simulink model "PID_simulink"  (R2018a)
settings: Solver=FixedStepAuto  StartTime=0.0  StopTime=t_end  FixedStep=0.0001  MinStep=1e-4  RelTol=1e-3
values from neighbouring files (symbols this model uses):
  Den = [1 12 24]    [PID.m]
  Kd = 3    [PID.m]
  Ki = 70    [PID.m]
  Kp = 50    [PID.m]
  Num = [2]    [PID.m]
settings Model: Creator=Milosh Yokich  LastModifiedBy=Milosh Yokich

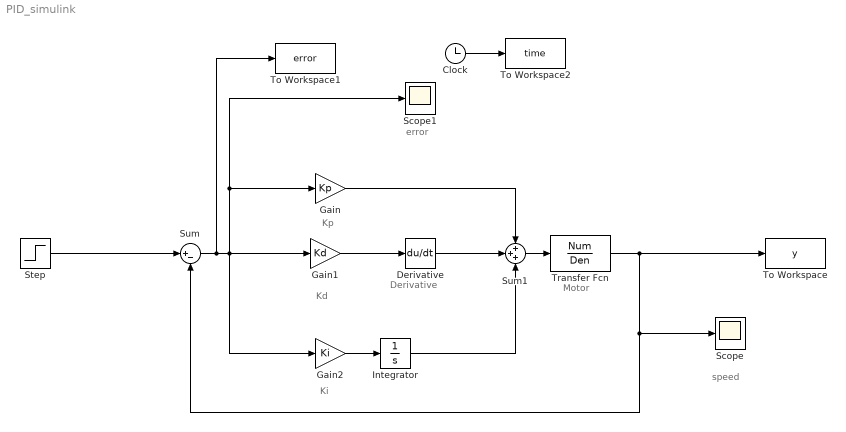
== system PID_simulink ==
  note: Ki
  note: error
  note: speed
  note: Derivative
  note: Motor
  note: Kd
  note: Kp
  Clock : Clock
  Derivative : Derivative  CoefficientInTFapproximation=0.000000000001
  Gain : Gain  Gain=Kp
  Gain1 : Gain  Gain=Kd
  Gain2 : Gain  Gain=Ki
  Integrator : Integrator  AbsoluteTolerance=1e-4
  Scope : Scope
  Scope1 : Scope
  Step : Step  Time=0  SampleTime=0
  Sum : Sum  Inputs=|+-
  Sum1 : Sum  Inputs=+++
  To Workspace : ToWorkspace  VariableName=y  SampleTime=-1
  To Workspace1 : ToWorkspace  VariableName=error  SampleTime=-1
  To Workspace2 : ToWorkspace  VariableName=time  SampleTime=-1
  Transfer Fcn : TransferFcn  Numerator=Num  Denominator=Den
  wires:
  Step/1 -> Sum/1
  Gain1/1 -> Derivative/1
  Derivative/1 -> Sum1/2
  Clock/1 -> To Workspace2/1
  Transfer Fcn/1 -> To Workspace/1, Scope/1, Sum/2
  Gain2/1 -> Integrator/1
  Integrator/1 -> Sum1/3
  Sum1/1 -> Transfer Fcn/1
  Gain/1 -> Sum1/1
  Sum/1 -> Gain2/1, Gain/1, Scope1/1, Gain1/1, To Workspace1/1
